simulink model "projeto_passa_alta"  (R2016a)
settings: Solver=ode23tb  StartTime=0.0  StopTime=10  MaxStep=1e-4  RelTol=1e-3
undefined symbols (not defined in the file or in its folder): C, L, R
libraries: powerlib x8
settings Model: Creator=renat  LastModifiedBy=renat

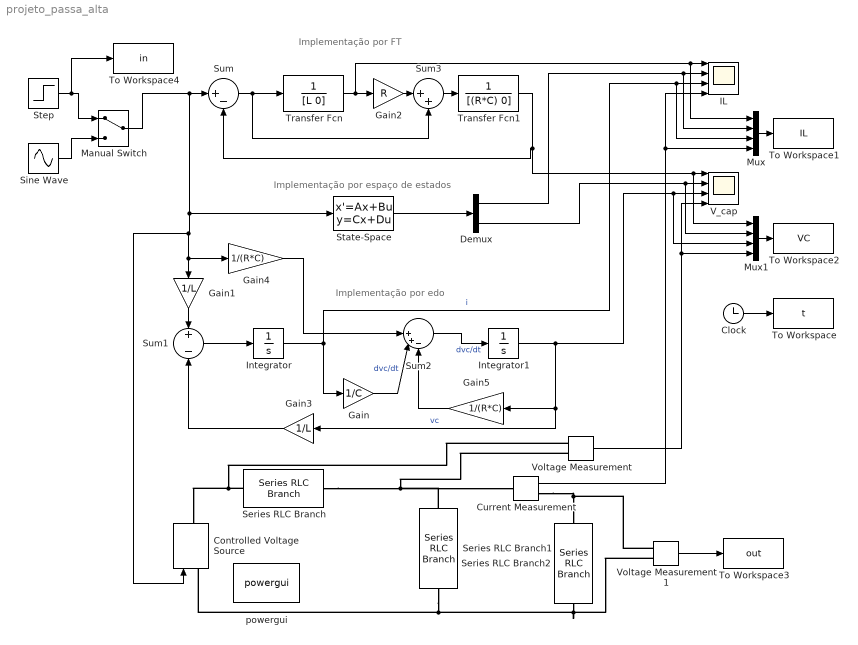
== system projeto_passa_alta ==
  note: Implementação por edo
  note: Implementação por espaço de estados
  note: Implementação por FT
  Clock : Clock
  Controlled Voltage Source : powerlib/Electrical Sources/Controlled Voltage Source  Initialize=on  Source_Type=AC  Amplitude=0  Phase=0  Frequency=0  Measurements=None
  Current Measurement : powerlib/Measurements/Current Measurement  PhasorSimulation=off  OutputType=Complex  PSBequivalent=0
  Demux : Demux  Outputs=2
  Gain : Gain  Gain=1/C
  Gain1 : Gain  Gain=1/L
  Gain2 : Gain  Gain=R
  Gain3 : Gain  Gain=1/L
  Gain4 : Gain  Gain=1/(R*C)
  Gain5 : Gain  Gain=1/(R*C)
  IL : Scope  NumInputPorts=4
  Integrator : Integrator
  Integrator1 : Integrator
  Manual Switch : ManualSwitch
  Mux : Mux
  Mux1 : Mux
  Series RLC Branch : powerlib/Elements/Series RLC Branch  LConnTagsString=__new0  RConnTagsString=__new0  BranchType=C  Resistance=R  Inductance=1e-3  SetiL0=off  InitialCurrent=0  Capacitance=C  Setx0=off  InitialVoltage=0  Measurements=None
  Series RLC Branch1 : powerlib/Elements/Series RLC Branch  LConnTagsString=__new0  RConnTagsString=__new0  BranchType=R  Resistance=R  Inductance=L  SetiL0=off  InitialCurrent=0  Capacitance=1e-6  Setx0=off  InitialVoltage=0  Measurements=None
  Series RLC Branch2 : powerlib/Elements/Series RLC Branch  LConnTagsString=__new0  RConnTagsString=__new0  BranchType=L  Resistance=R  Inductance=L  SetiL0=off  InitialCurrent=0  Capacitance=C  Setx0=off  InitialVoltage=0  Measurements=None
  Sine Wave : Sin  Amplitude=10*sqrt(2)  Frequency=1000  SampleTime=0
  State-Space : StateSpace  A="[0 -1/L;1/C  -1/(R*C)]"  B=[1/L; 1/(R*C)]  C=[1 0; 0 1]  D=[0; 0]  X0=0
  Step : Step  Time=0  After=10  SampleTime=0
  Sum : Sum  Inputs=|+-
  Sum1 : Sum  Inputs=+-
  Sum2 : Sum  Inputs=||++-
  Sum3 : Sum  Inputs=|++
  To Workspace : ToWorkspace  VariableName=t  SampleTime=-1
  To Workspace1 : ToWorkspace  VariableName=IL  SampleTime=-1
  To Workspace2 : ToWorkspace  VariableName=VC  SampleTime=-1
  To Workspace3 : ToWorkspace  VariableName=out  SampleTime=-1
  To Workspace4 : ToWorkspace  VariableName=in  SampleTime=-1
  Transfer Fcn : TransferFcn  Denominator=[L 0]
  Transfer Fcn1 : TransferFcn  Denominator=[(R*C) 0]
  V_cap : Scope  NumInputPorts=4
  Voltage Measurement : powerlib/Measurements/Voltage Measurement  PhasorSimulation=off  OutputType=Complex  PSBequivalent=0
  Voltage Measurement1 : powerlib/Measurements/Voltage Measurement  PhasorSimulation=off  OutputType=Complex  PSBequivalent=0
  powergui : powerlib/powergui  Priority=1  SimulationMode=Continuous  SolverType=Tustin/Backward Euler (TBE)  SampleTime=50e-6  frequency=60  SPID=off  DisableSnubberDevices=off  DisableRonSwitches=off  DisableVfSwitches=off  SwTol=0  DisplayEquations=off  Interpol=off  ExternalGateDelay=off  methode=off  Ts=10  FunctionMessages=off  echomessages=off  HookPort=off  EnableUseOfTLC=off  x0status=blocks  frequencyindice=0  Pbase=100e6  ErrMax=1e-4  Iterations=50  UnitsV=kV  UnitsW=MW  buscounter=0  RestoreLinks=warning  ResistiveCurrentMeasurement=off  Frange=[0:2:500]  Ylog=off  Xlog=on  ShowGrid=off  save=off  variable=ZData  structure=0  ZoomFFT=off  StartTime=0.0  cycles=1  DisplayStyle=1  fundamental=60  FreqAxis=off  MaxFrequency=1000  frequencyindicesteady=1  RmsSteady=1  display=off
  wires:
  Manual Switch/1 -> Controlled Voltage Source/1, Gain1/1, Gain4/1, State-Space/1, Sum/1
  Sum/1 -> Sum3/2, Transfer Fcn/1
  Transfer Fcn/1 -> Gain2/1, Mux/1, IL/1
  Transfer Fcn1/1 -> Sum/2, Mux1/1, V_cap/1
  State-Space/1 -> Demux/1
  Demux/1 -> Mux/2, IL/2
  Demux/2 -> Mux1/2, V_cap/2
  Sum1/1 -> Integrator/1
  Gain1/1 -> Sum1/1
  Integrator/1 -> Mux/3, IL/3, Gain/1  "i"
  Gain3/1 -> Sum1/2
  Integrator1/1 -> Mux1/3, V_cap/3, Gain3/1, Gain5/1  "vc"
  Sum2/1 -> Integrator1/1  "dvc/dt"
  Current Measurement/1 -> IL/4, Mux/4
  Voltage Measurement/1 -> Mux1/4, V_cap/4
  Step/1 -> To Workspace4/1, Manual Switch/1
  Sine Wave/1 -> Manual Switch/2
  Voltage Measurement1/1 -> To Workspace3/1
  Gain/1 -> Sum2/2  "dvc/dt"
  Gain4/1 -> Sum2/1
  Gain5/1 -> Sum2/3
  Gain2/1 -> Sum3/1
  Sum3/1 -> Transfer Fcn1/1
  Clock/1 -> To Workspace/1
  Mux/1 -> To Workspace1/1
  Mux1/1 -> To Workspace2/1
  connections:
  Series RLC Branch/RConn1 -- Voltage Measurement/LConn2 -- Series RLC Branch1/LConn1 -- Current Measurement/LConn1
  Series RLC Branch/LConn1 -- Voltage Measurement/LConn1 -- Controlled Voltage Source/RConn1
  Current Measurement/RConn1 -- Voltage Measurement1/LConn1 -- Series RLC Branch2/LConn1
  Series RLC Branch2/RConn1 -- Series RLC Branch1/RConn1 -- Controlled Voltage Source/LConn1 -- Voltage Measurement1/LConn2
